simulink model "slave_task"  (Simulink 3.0)
libraries: mathlib x4, logiclib x2, inoutlib x2, reglib x2

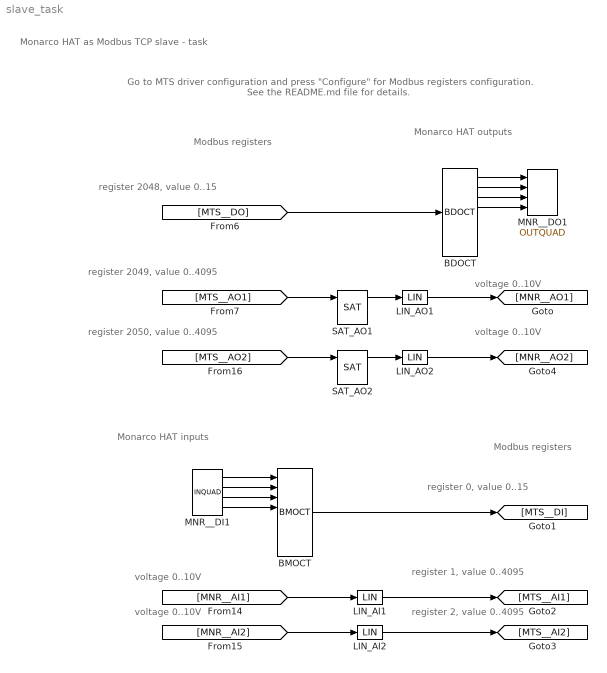
== system slave_task ==
  note: Modbus registers
  note: Modbus registers
  note: Go to MTS driver configuration and press "Configure" for Modbus registers configuration.
      |
      | See the README.md file for details.
  note: Monarco HAT as Modbus TCP slave - task
  note: Monarco HAT outputs
  note: register 2049, value 0..4095
  note: register 2050, value 0..4095
  note: Monarco HAT inputs
  note: register 2048, value 0..15
  note: register 0, value 0..15
  note: register 1, value 0..4095
  note: register 2, value 0..4095
  note: voltage 0..10V
  note: voltage 0..10V
  note: voltage 0..10V
  note: voltage 0..10V
  BDOCT : logiclib/BDOCT  shift=0
  BMOCT : logiclib/BMOCT  shift=0
  LIN_AI1 : mathlib/LIN  u1=0  y1=0  u2=10  y2=4095
  LIN_AI2 : mathlib/LIN  u1=0  y1=0  u2=10  y2=4095
  LIN_AO1 : mathlib/LIN  u1=0  y1=0  u2=4095  y2=10
  LIN_AO2 : mathlib/LIN  u1=0  y1=0  u2=4095  y2=10
  MNR__DI1 : inoutlib/INQUAD
  MNR__DO1 : inoutlib/OUTQUAD
  SAT_AO1 : reglib/SAT  tp=1  tn=1  hilim0=4095  lolim0=0  HLD=on
  SAT_AO2 : reglib/SAT  tp=1  tn=1  hilim0=4095  lolim0=0  HLD=on
  wires:
  BDOCT/1 -> MNR__DO1/1
  BDOCT/2 -> MNR__DO1/2
  BDOCT/3 -> MNR__DO1/3
  BDOCT/4 -> MNR__DO1/4
  BMOCT/1 -> [MTS__DI]
  [MNR__AI1] -> LIN_AI1/1
  [MNR__AI2] -> LIN_AI2/1
  [MTS__AO2] -> SAT_AO2/1
  [MTS__DO] -> BDOCT/1
  [MTS__AO1] -> SAT_AO1/1
  LIN_AI1/1 -> [MTS__AI1]
  LIN_AI2/1 -> [MTS__AI2]
  LIN_AO1/1 -> [MNR__AO1]
  LIN_AO2/1 -> [MNR__AO2]
  MNR__DI1/1 -> BMOCT/1
  MNR__DI1/2 -> BMOCT/2
  MNR__DI1/3 -> BMOCT/3
  MNR__DI1/4 -> BMOCT/4
  SAT_AO1/1 -> LIN_AO1/1
  SAT_AO2/1 -> LIN_AO2/1
